simulink model "full_dc_to_dc_bipo"  (R2018b)
settings: Solver=VariableStepAuto  StartTime=0.0  StopTime=5  MaxStep=1e-4  RelTol=1e-3
libraries: powerlib x15, powerlib_meascontrol x1
settings Model: Creator=Mohamad  LastModifiedBy=PARTO
settings SFSimCC: SimUseLocalCustomCode=off
settings RTWCC: RTWUseLocalCustomCode=off
settings CodeAppCC: StateflowObjectComments=on
settings SimscapeCC: SimscapeNormalizeSystem=off

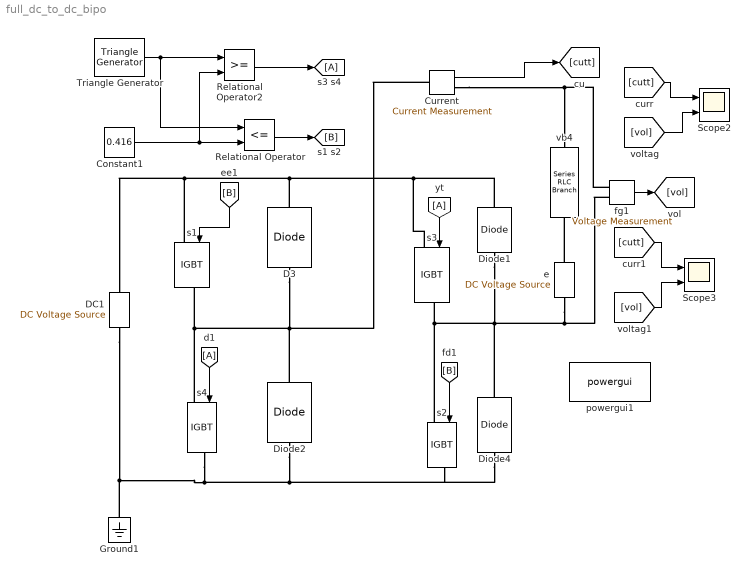
== system full_dc_to_dc_bipo ==
  Constant1 : Constant  Value=0.416
  Current : powerlib/Measurements/Current Measurement  PhasorSimulation=off  OutputType=Complex  PSBequivalent=0
      settings: SourceProductName=Simscape Electrical
  D3 : powerlib/Power Electronics/Diode  Ron=0.001  Lon=0  Vf=0.8  IC=0  UseSnubber=0  Rs=500  Cs=250e-9  Measurements=off
      settings: SourceProductName=Simscape Electrical
  DC1 : powerlib/Electrical Sources/DC Voltage Source  Amplitude=200  Measurements=None
      settings: SourceProductName=Simscape Electrical
  Diode1 : powerlib/Power Electronics/Diode  Ron=0.001  Lon=0  Vf=0.8  IC=0  UseSnubber=0  Rs=500  Cs=250e-9  Measurements=off
      settings: SourceProductName=Simscape Electrical
  Diode2 : powerlib/Power Electronics/Diode  Ron=0.001  Lon=0  Vf=0.8  IC=0  UseSnubber=0  Rs=500  Cs=250e-9  Measurements=off
      settings: SourceProductName=Simscape Electrical
  Diode4 : powerlib/Power Electronics/Diode  Ron=0.001  Lon=0  Vf=0.8  IC=0  UseSnubber=0  Rs=500  Cs=250e-9  Measurements=off
      settings: SourceProductName=Simscape Electrical
  Ground1 : powerlib/Elements/Ground  LConnTagsString=a
      settings: SourceProductName=Simscape Electrical
  Relational Operator : RelationalOperator  Operator=<=  OutDataTypeStr=boolean  RndMeth=Simplest
  Relational Operator2 : RelationalOperator  OutDataTypeStr=boolean  RndMeth=Simplest
  Scope2 : Scope  NumInputPorts=2
  Scope3 : Scope  NumInputPorts=2
  Triangle Generator : powerlib_meascontrol/Pulse & Signal Generators/Triangle Generator  Freq=1000  Phase=0  Ts=0
      settings: SourceProductName=Simscape Electrical
  e : powerlib/Electrical Sources/DC Voltage Source  Amplitude=2  Measurements=None
      settings: SourceProductName=Simscape Electrical
  fg1 : powerlib/Measurements/Voltage Measurement  PhasorSimulation=off  OutputType=Complex  PSBequivalent=0
      settings: SourceProductName=Simscape Electrical
  powergui1 : powerlib/powergui  Priority=1  SimulationMode=Continuous  SampleTime=50e-6  frequency=60  Iterations=50  frequencyindice=0  Pbase=100e6  ErrMax=1e-4  UnitsV=kV  UnitsW=MW  buscounter=0  FunctionMessages=off  echomessages=off  EnableUseOfTLC=off  CurrentSourceSwitches=off  DisableSnubberDevices=off  DisableRonSwitches=off  DisableVfSwitches=off  DisplayEquations=off  SolverType=Tustin/Backward Euler (TBE)  Interpol=off  ExternalGateDelay=off  methode=off  Ts=100  x0status=blocks  SPID=on  SwTol=0  HookPort=off  RestoreLinks=warning  ResistiveCurrentMeasurement=off  Frange=[0:2:500]  Ylog=off  Xlog=on  ShowGrid=off  save=off  variable=ZData  structure=0  ZoomFFT=off  StartTime=0.0  cycles=1  DisplayStyle=1  fundamental=60  FreqAxis=off  MaxFrequency=1000  frequencyindicesteady=1  RmsSteady=1  display=off
      settings: SourceProductName=Simscape Electrical
  s{1..4} (4 alike) : powerlib/Power Electronics/IGBT  Ron=0.001  Lon=0  Vf=1  Tf=1e-6  Tt=2e-6  IC=0  Rs=1e5  Cs=inf  Measurements=off
      settings: SourceProductName=Simscape Electrical
  vb4 : powerlib/Elements/Series RLC Branch  LConnTagsString=__new0  RConnTagsString=__new0  BranchType=RL  Resistance=0.5  Inductance=1  SetiL0=off  InitialCurrent=0  Capacitance=60e-6  Setx0=off  InitialVoltage=0  Measurements=None
      settings: SourceProductName=Simscape Electrical
  wires:
  Triangle Generator/1 -> Relational Operator/1, Relational Operator2/1
  [A] -> s3/1
  [B] -> s1/1
  [B] -> s2/1
  Relational Operator/1 -> [B]
  Constant1/1 -> Relational Operator2/2, Relational Operator/2
  [A] -> s4/1
  Relational Operator2/1 -> [A]
  fg1/1 -> [vol]
  Current/1 -> [cutt]
  [vol] -> Scope2/2
  [vol] -> Scope3/2
  [cutt] -> Scope2/1
  [cutt] -> Scope3/1
  connections:
  Current/RConn1 -- fg1/LConn1 -- vb4/LConn1
  fg1/LConn2 -- e/LConn1 -- Diode4/RConn1 -- Diode1/LConn1 -- s2/LConn1 -- s3/RConn1
  Ground1/LConn1 -- s4/RConn1 -- Diode4/LConn1 -- s2/RConn1 -- Diode2/LConn1 -- DC1/LConn1
  D3/LConn1 -- Diode2/RConn1 -- Current/LConn1 -- s4/LConn1 -- s1/RConn1
  s3/LConn1 -- Diode1/RConn1 -- D3/RConn1 -- DC1/RConn1 -- s1/LConn1
  e/RConn1 -- vb4/RConn1
